simulink model "simu_lin_bouclage_1rob"  (Simulink 7.5)
settings: Solver=ode3  StartTime=0.0  StopTime=3  FixedStep=0.02  RelTol=1e-3
libraries: simulink x2, simulink_need_slupdate x2
settings Model: Creator=FClaveau  LastModifiedBy=fclaveau
settings DebuggingCC: SaveWithParameterizedLinksMsg=none  MultiTaskCondExecSysMsg=none  StrictBusMsg=Warning
settings RTWCC: IncludeERTFirstTime=on

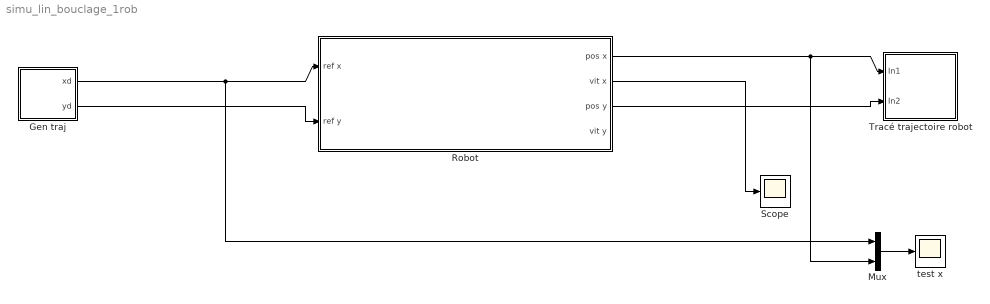
== system simu_lin_bouclage_1rob ==
  Gen traj : Subsystem
  Mux : Mux  Inputs=2
  Robot : Subsystem
  Scope : Scope
  Tracé trajectoire robot : Subsystem
  test x : Scope
      settings: YMin=0  YMax=15  SaveName=ScopeData2
  wires:
  Gen traj/1(xd) -> Robot/1(ref x), Mux/1
  Gen traj/2(yd) -> Robot/2(ref y)
  Robot/1(pos x) -> Tracé trajectoire robot/1(In1), Mux/2
  Robot/3(pos y) -> Tracé trajectoire robot/2(In2)
  Robot/2(vit x) -> Scope/1
  Mux/1 -> test x/1

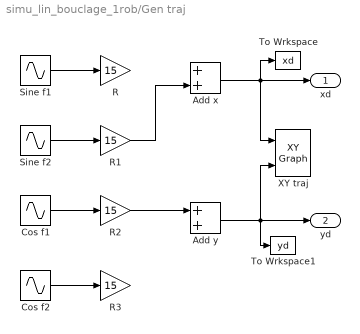
== system simu_lin_bouclage_1rob/Gen traj ==
  Add x : Sum  OutDataType=fixdt(1, 16)  OutScaling=2^-10
  Add y : Sum  OutDataType=fixdt(1, 16)  OutScaling=2^-10
  Cos f1 : Sin  Amplitude=1  Bias=0  Frequency=2/2/pi  Phase=0  Samples=10  SampleTime=0  Offset=0
  Cos f2 : Sin  Amplitude=1  Bias=0  Frequency=12/2/pi  Phase=0  Samples=10  SampleTime=0  Offset=0
  R{,1..3} (4 alike) : Gain  Gain=15  ParameterDataType=fixdt(1, 16)  ParameterScaling=2^0  OutDataType=fixdt(1, 16)  OutScaling=2^0
  Sine f1 : Sin  Amplitude=1  Bias=0  Frequency=2/2/pi  Phase=0  Samples=10  SampleTime=0  Offset=0
  Sine f2 : Sin  Amplitude=1  Bias=0  Frequency=12/2/pi  Phase=0  Samples=10  SampleTime=0  Offset=0
  To Wrkspace : ToWorkspace  VariableName=xd  SampleTime=-1  SaveFormat=Structure
  To Wrkspace1 : ToWorkspace  VariableName=yd  SampleTime=-1  SaveFormat=Structure
  XY traj : simulink/Sinks/XY Graph  SystemSampleTime=-1  xmin=-20  xmax=20  ymin=-20  ymax=20  st=-1
  xd : Outport
  yd : Outport  Port=2
  wires:
  Sine f1/1 -> R/1
  Sine f2/1 -> R1/1
  Cos f1/1 -> R2/1
  Cos f2/1 -> R3/1
  R1/1 -> Add x/2
  R2/1 -> Add y/1
  Add x/1 -> xd/1, To Wrkspace/1, XY traj/1
  Add y/1 -> yd/1, To Wrkspace1/1, XY traj/2

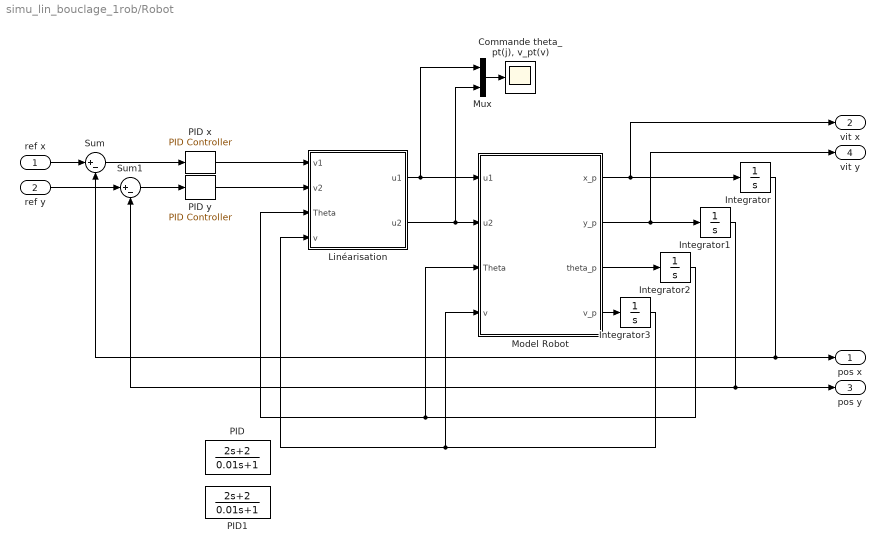
== system simu_lin_bouclage_1rob/Robot ==
  ref x : Inport
  ref y : Inport  Port=2
  "Commande theta_pt(j), v_pt(v)" : Scope
  Integrator : Integrator
  Integrator1 : Integrator
  Integrator2 : Integrator  InitialCondition=1
  Integrator3 : Integrator  InitialCondition=2
  Linéarisation : Subsystem
  Model Robot : Subsystem
  Mux : Mux  Inputs=2
  PID : TransferFcn  Numerator=[2 2]  Denominator=[0.01 1]
  PID x : simulink_need_slupdate/PID Controller  SystemSampleTime=-1  P=2  I=0  D=2
  PID y : simulink_need_slupdate/PID Controller  SystemSampleTime=-1  P=2  I=0  D=2
  PID1 : TransferFcn  Numerator=[2 2]  Denominator=[0.01 1]
  Sum : Sum  Inputs=|+-  OutDataType=fixdt(1, 16)  OutScaling=2^0
  Sum1 : Sum  Inputs=|+-  OutDataType=fixdt(1, 16)  OutScaling=2^0
  pos x : Outport
  vit x : Outport  Port=2
  pos y : Outport  Port=3
  vit y : Outport  Port=4
  wires:
  Model Robot/1(x_p) -> Integrator/1, vit x/1
  Model Robot/2(y_p) -> Integrator1/1, vit y/1
  Model Robot/3(theta_p) -> Integrator2/1
  Model Robot/4(v_p) -> Integrator3/1
  Integrator2/1 -> Model Robot/3(Theta), Linéarisation/3(Theta)
  Integrator3/1 -> Model Robot/4(v), Linéarisation/4(v)
  PID x/1 -> Linéarisation/1(v1)
  PID y/1 -> Linéarisation/2(v2)
  Sum/1 -> PID x/1
  Integrator/1 -> Sum/2, pos x/1
  Sum1/1 -> PID y/1
  Integrator1/1 -> Sum1/2, pos y/1
  Linéarisation/1(u1) -> Model Robot/1(u1), Mux/1
  Linéarisation/2(u2) -> Model Robot/2(u2), Mux/2
  Mux/1 -> "Commande theta_pt(j), v_pt(v)"/1
  ref x/1 -> Sum/1
  ref y/1 -> Sum1/1

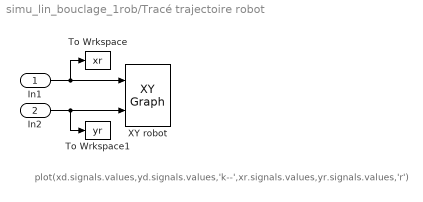
== system simu_lin_bouclage_1rob/Tracé trajectoire robot ==
  note: plot(xd.signals.values,yd.signals.values,'k--',xr.signals.values,yr.signals.values,'r')
  In1 : Inport  OutDataType=sfix(16)  OutScaling=2^0
  In2 : Inport  Port=2  OutDataType=sfix(16)  OutScaling=2^0
  To Wrkspace : ToWorkspace  VariableName=xr  SampleTime=-1  SaveFormat=Structure
  To Wrkspace1 : ToWorkspace  VariableName=yr  SampleTime=-1  SaveFormat=Structure
  XY robot : simulink/Sinks/XY Graph  SystemSampleTime=-1  xmin=-20  xmax=20  ymin=-20  ymax=20  st=-1
  wires:
  In1/1 -> XY robot/1, To Wrkspace/1
  In2/1 -> XY robot/2, To Wrkspace1/1

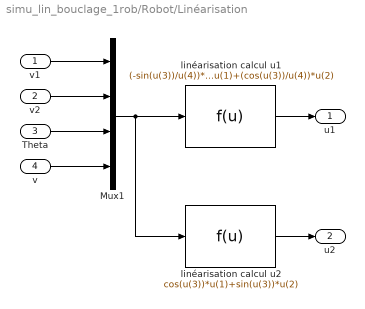
== system simu_lin_bouclage_1rob/Robot/Linéarisation ==
  v1 : Inport
  v2 : Inport  Port=2
  Theta : Inport  Port=3
  v : Inport  Port=4
  Mux1 : Mux
  linéarisation calcul u1 : Fcn  Expr=(-sin(u(3))/u(4))*u(1)+(cos(u(3))/u(4))*u(2)
  linéarisation calcul u2 : Fcn  Expr=cos(u(3))*u(1)+sin(u(3))*u(2)
  u1 : Outport
  u2 : Outport  Port=2
  wires:
  v1/1 -> Mux1/1
  v2/1 -> Mux1/2
  Theta/1 -> Mux1/3
  v/1 -> Mux1/4
  Mux1/1 -> linéarisation calcul u1/1, linéarisation calcul u2/1
  linéarisation calcul u2/1 -> u2/1
  linéarisation calcul u1/1 -> u1/1

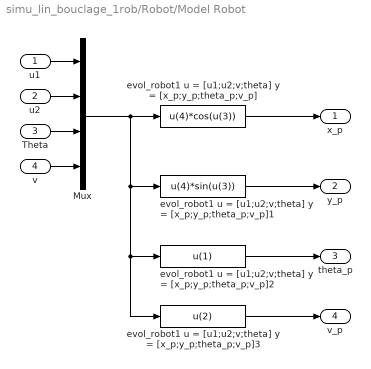
== system simu_lin_bouclage_1rob/Robot/Model Robot ==
  u1 : Inport
  u2 : Inport  Port=2
  Theta : Inport  Port=3
  v : Inport  Port=4
  Mux : Mux
  evol_robot1 u = [u1;u2;v;theta] y = [x_p;y_p;theta_p;v_p] : Fcn  Expr=u(4)*cos(u(3))
  evol_robot1 u = [u1;u2;v;theta] y = [x_p;y_p;theta_p;v_p]1 : Fcn  Expr=u(4)*sin(u(3))
  evol_robot1 u = [u1;u2;v;theta] y = [x_p;y_p;theta_p;v_p]2 : Fcn  Expr=u(1)
  evol_robot1 u = [u1;u2;v;theta] y = [x_p;y_p;theta_p;v_p]3 : Fcn  Expr=u(2)
  x_p : Outport
  y_p : Outport  Port=2
  theta_p : Outport  Port=3
  v_p : Outport  Port=4
  wires:
  evol_robot1 u = [u1;u2;v;theta] y = [x_p;y_p;theta_p;v_p]/1 -> x_p/1
  Mux/1 -> evol_robot1 u = [u1;u2;v;theta] y = [x_p;y_p;theta_p;v_p]/1, evol_robot1 u = [u1;u2;v;theta] y = [x_p;y_p;theta_p;v_p]1/1, evol_robot1 u = [u1;u2;v;theta] y = [x_p;y_p;theta_p;v_p]2/1, evol_robot1 u = [u1;u2;v;theta] y = [x_p;y_p;theta_p;v_p]3/1
  u1/1 -> Mux/1
  u2/1 -> Mux/2
  Theta/1 -> Mux/3
  v/1 -> Mux/4
  evol_robot1 u = [u1;u2;v;theta] y = [x_p;y_p;theta_p;v_p]1/1 -> y_p/1
  evol_robot1 u = [u1;u2;v;theta] y = [x_p;y_p;theta_p;v_p]2/1 -> theta_p/1
  evol_robot1 u = [u1;u2;v;theta] y = [x_p;y_p;theta_p;v_p]3/1 -> v_p/1
